simulink model "JT_60SA_scheme_nov_2017_RU_2015a"  (R2015b)
settings: Solver=ode45  SolverMode=SingleTasking  StartTime=startTime-neg_time  StopTime=stopTime  RelTol=1e-5
values from neighbouring files (symbols this model uses):
  A_contr = A    [JT_60SA_simulator_VS_SOF18d66_japs_sensors_adriano_isoflux.m]    (also in JT_60SA_simulator_VS_SOF18d66_japs_sensors_isoflux_sqzd.m)
  B_contr = [B(:,[1:12 end]) A_contr*E]    [JT_60SA_simulator_VS_SOF18d66_japs_sensors_adriano_isoflux.m]    (also in JT_60SA_simulator_VS_SOF18d66_japs_sensors_isoflux_sqzd.m)
  C_contr = LinearModel.C(outputIdx,:)    [JT_60SA_simulator_VS_SOF18d66_japs_sensors_adriano_isoflux.m]    (also in JT_60SA_simulator_VS_SOF18d66_japs_sensors_isoflux_sqzd.m)
  CSsat = [1 1.3 1.3 1] * 1e3    [JT_60SA_simulator_VS_SOF18d66_japs_sensors_adriano_isoflux.m]    (also in JT_60SA_simulator_VS_SOF18d66_japs_sensors_isoflux_sqzd.m)
  D_contr = [LinearModel.D(outputIdx,[1:12 end]) LinearModel.F(outputIdx,:)+C_contr*E]    [JT_60SA_simulator_VS_SOF18d66_japs_sensors_adriano_isoflux.m]    (also in JT_60SA_simulator_VS_SOF18d66_japs_sensors_isoflux_sqzd.m)
  EFsat = [1 .97 .97 .97 .97 1] * 1e3    [JT_60SA_simulator_VS_SOF18d66_japs_sensors_adriano_isoflux.m]    (also in JT_60SA_simulator_VS_SOF18d66_japs_sensors_isoflux_sqzd.m)
  equilDist = LinearModel.YEquil(LinearModel.DisturbancesInfo.OutputPosition)    [JT_60SA_simulator_VS_SOF18d66_japs_sensors_adriano_isoflux.m]    (also in JT_60SA_simulator_VS_SOF18d66_japs_sensors_isoflux_sqzd.m)
  equilOutputs = LinearModel.YEquil(outputIdx)    [JT_60SA_simulator_VS_SOF18d66_japs_sensors_adriano_isoflux.m]    (also in JT_60SA_simulator_VS_SOF18d66_japs_sensors_isoflux_sqzd.m)
  equilVolts = zeros(13,1)    [JT_60SA_simulator_VS_SOF18d66_japs_sensors_adriano_isoflux.m]    (also in JT_60SA_simulator_VS_SOF18d66_japs_sensors_isoflux_sqzd.m)
  I_sat_lower = [-2 -2 -2 -2 -2 -2 -2 -2 -2 -2]*1e4    [JT_60SA_simulator_VS_SOF18d66_japs_sensors_adriano_isoflux.m]    (also in JT_60SA_simulator_VS_SOF18d66_japs_sensors_isoflux_sqzd.m)
  I_sat_upper = [2 2 2 2 1 1 2 2 1 1]*1e4    [JT_60SA_simulator_VS_SOF18d66_japs_sensors_adriano_isoflux.m]    (also in JT_60SA_simulator_VS_SOF18d66_japs_sensors_isoflux_sqzd.m)
  kIp = kIp/norm(kIp)    [JT_60SA_simulator_VS_SOF18d66_japs_sensors_adriano_isoflux.m]    (also in JT_60SA_simulator_VS_SOF18d66_japs_sensors_isoflux_sqzd.m)
  nOfGaps = 85    [JT_60SA_simulator_VS_SOF18d66_japs_sensors_adriano_isoflux.m]    (also in JT_60SA_simulator_VS_SOF18d66_japs_sensors_isoflux_sqzd.m)
  nOfStrikes = 8    [JT_60SA_simulator_VS_SOF18d66_japs_sensors_adriano_isoflux.m]    (also in JT_60SA_simulator_VS_SOF18d66_japs_sensors_isoflux_sqzd.m)
  PSdelay = 1.5e-3    (= 0.0015)    [JT_60SA_simulator_VS_SOF18d66_japs_sensors_adriano_isoflux.m]    (also in JT_60SA_simulator_VS_SOF18d66_japs_sensors_isoflux_sqzd.m)
  PSmodel = tf([1],[PStau 1]) * eye(nPF)    [JT_60SA_simulator_VS_SOF18d66_japs_sensors_adriano_isoflux.m]    (also in JT_60SA_simulator_VS_SOF18d66_japs_sensors_isoflux_sqzd.m)
  vLoop = LinearModel.R(end,end)*Ip0    [JT_60SA_simulator_VS_SOF18d66_japs_sensors_adriano_isoflux.m]    (also in JT_60SA_simulator_VS_SOF18d66_japs_sensors_isoflux_sqzd.m)
  xi0 = zeros(1, size(A_contr, 1))    [JT_60SA_simulator_VS_SOF18d66_japs_sensors_adriano_isoflux.m]    (also in JT_60SA_simulator_VS_SOF18d66_japs_sensors_isoflux_sqzd.m)
  XSC_matrix = XSC_matrix(:, 1:end-1)    [XSC_adriano_isoflux.m]
undefined symbols (not defined in the file or in its folder): KPFcurr, VS
libraries: cstblocks x5
settings Model: Creator=Adriano  LastModifiedBy=Dom
settings DataIOCC: SaveFormat=Array
settings OptimizationCC: BlockReduction=off  BooleanDataType=off
settings DebuggingCC: SaveWithParameterizedLinksMsg=none  UnderspecifiedInitializationDetection=Classic  MergeDetectMultiDrivingBlocksExec=none  SignalResolutionControl=TryResolveAllWithWarning
settings HardwareCC: ProdBitPerPointer=32  ProdLargestAtomicFloat=None  ProdIntDivRoundTo=Undefined  ProdEndianess=Unspecified  ProdWordSize=32  ProdHWDeviceType=32-bit Generic  TargetUnknown=on
settings GRTTargetCC: GeneratePreprocessorConditionals=Disable all
settings ConfigComp: CovModelRefEnable=Off

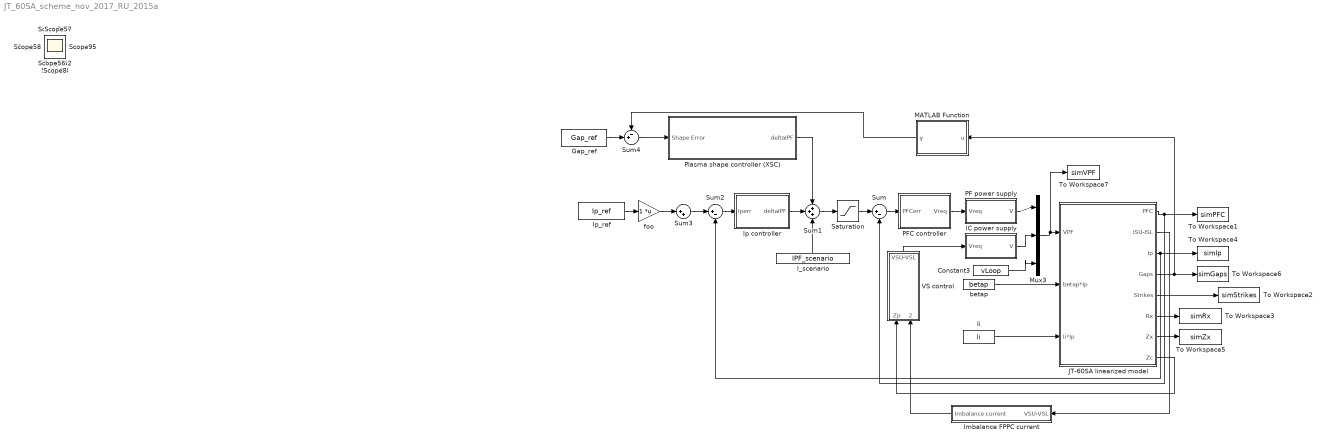
== system JT_60SA_scheme_nov_2017_RU_2015a ==
  Constant3 : Constant  Value=vLoop
  Gap_ref : FromWorkspace  VariableName=Gap_ref  SampleTime=0  OutputAfterFinalValue=Holding final value
  IC power supply : Subsystem
  I_scenario : FromWorkspace  VariableName=IPF_scenario  SampleTime=0  OutputAfterFinalValue=Holding final value
  Imbalance FPPC current : Subsystem
  Ip controller : Subsystem
  Ip_ref : FromWorkspace  VariableName=Ip_ref  SampleTime=0  OutputAfterFinalValue=Holding final value
  JT-60SA linearized model : Subsystem
  MATLAB Function : MATLAB Function  TreatAsAtomicUnit=on
  Mux3 : Mux  Inputs=3
  PF power supply : Subsystem
  PFC controller : Subsystem
  Plasma shape controller (XSC) : Subsystem
  Saturation : Saturate  UpperLimit=I_sat_upper  LowerLimit=I_sat_lower
  Sum : Sum  Inputs=|+-
  Sum1 : Sum  Inputs=+++
  Sum2 : Sum  Inputs=|+-
  Sum3 : Sum  Inputs=|++
  Sum4 : Sum  Inputs=-+|
  To Workspace1 : ToWorkspace  VariableName=simPFC  SaveFormat=Structure With Time  SampleTime=-1
  To Workspace2 : ToWorkspace  VariableName=simStrikes  SaveFormat=Structure With Time  SampleTime=-1
  To Workspace3 : ToWorkspace  VariableName=simRx  SaveFormat=Structure With Time  SampleTime=-1
  To Workspace4 : ToWorkspace  VariableName=simIp  SaveFormat=Structure With Time  SampleTime=-1
  To Workspace5 : ToWorkspace  VariableName=simZx  SaveFormat=Structure With Time  SampleTime=-1
  To Workspace6 : ToWorkspace  VariableName=simGaps  SaveFormat=Structure With Time  SampleTime=-1
  To Workspace7 : ToWorkspace  VariableName=simVPF  SaveFormat=Structure With Time  SampleTime=-1
  VS control : Subsystem
  betap : FromWorkspace  VariableName=betap  SampleTime=0  OutputAfterFinalValue=Holding final value
  foo : Gain  Multiplication=Matrix(K*u)
  li : FromWorkspace  VariableName=li  SampleTime=0  OutputAfterFinalValue=Holding final value
  Scope{,1..58} (59 alike) : Scope
  wires:
  li/1 -> JT-60SA linearized model/3(li*Ip)
  betap/1 -> JT-60SA linearized model/2(betap*Ip)
  JT-60SA linearized model/1(PFC) -> Sum/2, To Workspace1/1
  Mux3/1 -> To Workspace7/1, JT-60SA linearized model/1(VPF)
  Constant3/1 -> Mux3/3
  JT-60SA linearized model/3(Ip) -> To Workspace4/1, Sum2/2
  JT-60SA linearized model/4(Gaps) -> To Workspace6/1, MATLAB Function/1(u)
  JT-60SA linearized model/5(Strikes) -> To Workspace2/1
  JT-60SA linearized model/6(Rx) -> To Workspace3/1
  JT-60SA linearized model/7(Zx) -> To Workspace5/1
  Sum1/1 -> Saturation/1
  PF power supply/1(V) -> Mux3/1
  PFC controller/1(Vreq) -> PF power supply/1(Vreq)
  Sum2/1 -> Ip controller/1(Iperr)
  Sum3/1 -> Sum2/1
  Ip_ref/1 -> foo/1
  foo/1 -> Sum3/1
  Sum4/1 -> Plasma shape controller (XSC)/1(Shape Error)
  Sum/1 -> PFC controller/1(PFCerr)
  Ip controller/1(deltaIPF) -> Sum1/2
  Saturation/1 -> Sum/1
  IC power supply/1(V) -> Mux3/2
  JT-60SA linearized model/8(Zc) -> VS control/1(Zp)
  JT-60SA linearized model/2(ISU-ISL) -> Imbalance FPPC current/1(VSU-VSL)
  Imbalance FPPC current/1(Imbalance current) -> VS control/2(VSU-VSL current)
  VS control/1(VSU-VSL) -> IC power supply/1(Vreq)
  Gap_ref/1 -> Sum4/2
  I_scenario/1 -> Sum1/3
  MATLAB Function/1(y) -> Sum4/1
  Plasma shape controller (XSC)/1(deltaIPF) -> Sum1/1

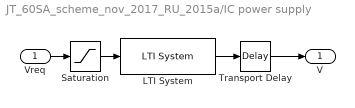
== system JT_60SA_scheme_nov_2017_RU_2015a/IC power supply ==
  Vreq : Inport
  LTI System : cstblocks/LTI System  sys=PSmodel(1:2, 1:2)  IC=[]
  Saturation : Saturate  UpperLimit=[1e3 1e3]  LowerLimit=[-1e3 -1e3]
  Transport Delay : TransportDelay  DelayTime=PSdelay
  V : Outport
  wires:
  LTI System/1 -> Transport Delay/1
  Vreq/1 -> Saturation/1
  Transport Delay/1 -> V/1
  Saturation/1 -> LTI System/1

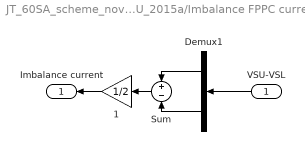
== system JT_60SA_scheme_nov_2017_RU_2015a/Imbalance FPPC current ==
  VSU-VSL : Inport
  "    1" : Gain  Gain=1/2
  Demux1 : Demux  Outputs=2
  Sum : Sum  Inputs=+|-
  Imbalance current : Outport
  wires:
  VSU-VSL/1 -> Demux1/1
  "    1"/1 -> Imbalance current/1
  Demux1/2 -> Sum/2
  Sum/1 -> "    1"/1
  Demux1/1 -> Sum/1

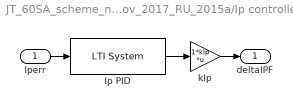
== system JT_60SA_scheme_nov_2017_RU_2015a/Ip controller ==
  Iperr : Inport
  Ip PID : cstblocks/LTI System  sys=Ip_PID  IC=[]
  kIp : Gain  Gain=1*kIp  Multiplication=Matrix(K*u)
  deltaIPF : Outport
  wires:
  Ip PID/1 -> kIp/1
  Iperr/1 -> Ip PID/1
  kIp/1 -> deltaIPF/1

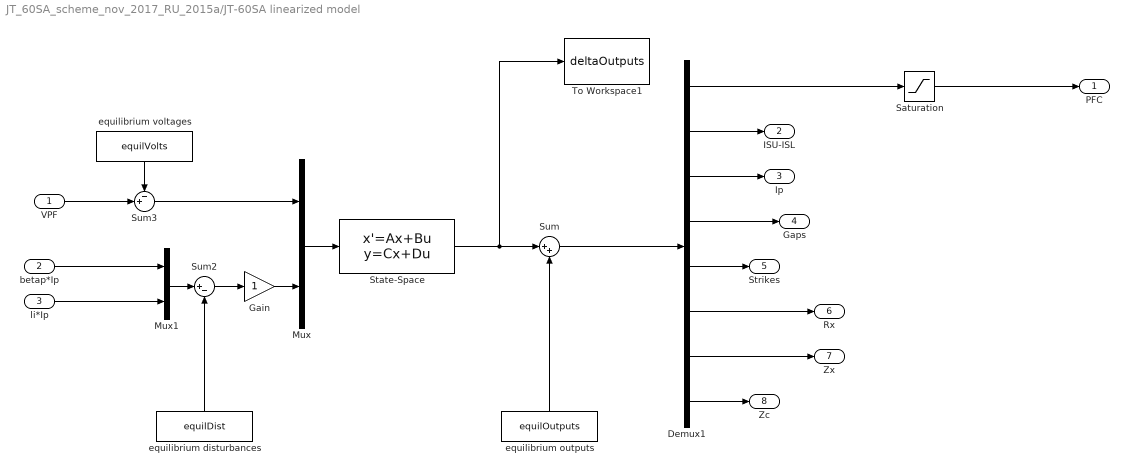
== system JT_60SA_scheme_nov_2017_RU_2015a/JT-60SA linearized model ==
  VPF : Inport
  betap*Ip : Inport  Port=2
  li*Ip : Inport  Port=3
  Demux1 : Demux  Outputs=[10 2 1 nOfGaps nOfStrikes 1 1 1]
  Gain : Gain
  Mux : Mux  Inputs=2
  Mux1 : Mux  Inputs=2
  Saturation : Saturate  UpperLimit=I_sat_upper  LowerLimit=I_sat_lower
  State-Space : StateSpace  A=A_contr  B=B_contr  C=C_contr  D=D_contr  X0=xi0
  Sum : Sum  Inputs=|++
  Sum2 : Sum  Inputs=|+-
  Sum3 : Sum  Inputs=-+|
  To Workspace1 : ToWorkspace  VariableName=deltaOutputs  SaveFormat=Structure With Time  SampleTime=-1
  equilibrium disturbances : Constant  Value=equilDist
  equilibrium outputs : Constant  Value=equilOutputs
  equilibrium voltages : Constant  Value=equilVolts
  PFC : Outport
  ISU-ISL : Outport  Port=2
  Ip : Outport  Port=3
  Gaps : Outport  Port=4
  Strikes : Outport  Port=5
  Rx : Outport  Port=6
  Zx : Outport  Port=7
  Zc : Outport  Port=8
  wires:
  State-Space/1 -> To Workspace1/1, Sum/1
  Sum/1 -> Demux1/1
  equilibrium outputs/1 -> Sum/2
  Mux/1 -> State-Space/1
  VPF/1 -> Sum3/2
  Demux1/1 -> Saturation/1
  Mux1/1 -> Sum2/1
  equilibrium disturbances/1 -> Sum2/2
  betap*Ip/1 -> Mux1/1
  li*Ip/1 -> Mux1/2
  Sum3/1 -> Mux/1
  equilibrium voltages/1 -> Sum3/1
  Sum2/1 -> Gain/1
  Demux1/3 -> Ip/1
  Demux1/4 -> Gaps/1
  Demux1/5 -> Strikes/1
  Demux1/6 -> Rx/1
  Demux1/7 -> Zx/1
  Gain/1 -> Mux/2
  Saturation/1 -> PFC/1
  Demux1/2 -> ISU-ISL/1
  Demux1/8 -> Zc/1

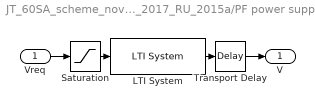
== system JT_60SA_scheme_nov_2017_RU_2015a/PF power supply ==
  Vreq : Inport
  LTI System : cstblocks/LTI System  sys=PSmodel  IC=[]
  Saturation : Saturate  UpperLimit=[CSsat EFsat]  LowerLimit=-[CSsat EFsat]
  Transport Delay : TransportDelay  DelayTime=PSdelay
  V : Outport
  wires:
  LTI System/1 -> Transport Delay/1
  Vreq/1 -> Saturation/1
  Transport Delay/1 -> V/1
  Saturation/1 -> LTI System/1

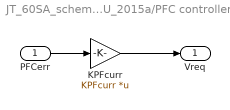
== system JT_60SA_scheme_nov_2017_RU_2015a/PFC controller ==
  PFCerr : Inport
  KPFcurr : Gain  Gain=KPFcurr  Multiplication=Matrix(K*u)
  Vreq : Outport
  wires:
  KPFcurr/1 -> Vreq/1
  PFCerr/1 -> KPFcurr/1

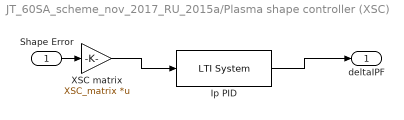
== system JT_60SA_scheme_nov_2017_RU_2015a/Plasma shape controller (XSC) ==
  Shape Error : Inport
  Ip PID : cstblocks/LTI System  sys=XSC_PI  IC=[]
  XSC matrix : Gain  Gain=XSC_matrix  Multiplication=Matrix(K*u)
  deltaIPF : Outport
  wires:
  Shape Error/1 -> XSC matrix/1
  XSC matrix/1 -> Ip PID/1
  Ip PID/1 -> deltaIPF/1

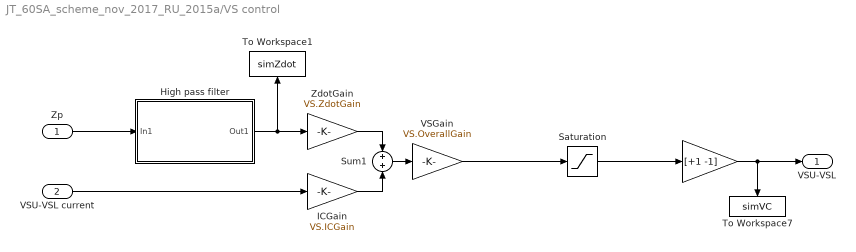
== system JT_60SA_scheme_nov_2017_RU_2015a/VS control ==
  Zp : Inport
  VSU-VSL current : Inport  Port=2
  "    " : Gain  Gain=[+1 -1]
  High pass filter : Subsystem
  ICGain : Gain  Gain=VS.ICGain
  Saturation : Saturate  UpperLimit=1e3  LowerLimit=-1e3
  Sum1 : Sum  Inputs=+|+
  To Workspace1 : ToWorkspace  VariableName=simZdot  SaveFormat=Structure With Time  SampleTime=-1
  To Workspace7 : ToWorkspace  VariableName=simVC  SaveFormat=Structure With Time  SampleTime=-1
  VSGain : Gain  Gain=VS.OverallGain
  ZdotGain : Gain  Gain=VS.ZdotGain
  VSU-VSL : Outport
  wires:
  VSU-VSL current/1 -> ICGain/1
  High pass filter/1(Out1) -> To Workspace1/1, ZdotGain/1
  Zp/1 -> High pass filter/1(In1)
  Sum1/1 -> VSGain/1
  ZdotGain/1 -> Sum1/1
  ICGain/1 -> Sum1/2
  "    "/1 -> VSU-VSL/1, To Workspace7/1
  VSGain/1 -> Saturation/1
  Saturation/1 -> "    "/1

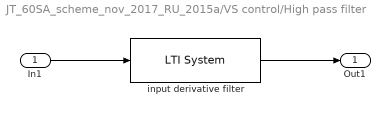
== system JT_60SA_scheme_nov_2017_RU_2015a/VS control/High pass filter ==
  In1 : Inport
  input derivative filter : cstblocks/LTI System  sys=VS.Filter  IC=[]
  Out1 : Outport
  wires:
  input derivative filter/1 -> Out1/1
  In1/1 -> input derivative filter/1

== matlab function JT_60SA_scheme_nov_2017_RU_2015a/MATLAB Function ==
  data: u input; y output
function y = fcn(u)
%#codegen
% % % %%all gaps
% y=u(1:end);

% %%30 gaps
%  y=u([1:3:(end-2),end-1,end]);
    
% %%19 gaps
%  y=u([1:5:(end-2),end-1,end]);

%20 gaps
 y=u([round((1+1:4.6:(end-2))),end-1,end]);

% % % Japanese selection1
% japs_gaps=[13,22,36,52,66,76,84,85  ]';
%  y=u(japs_gaps);
% % % % % % 
% % % %Japanese selection 2
%  japs_gaps=[21,36,47,66,84,85]';
% y=u(japs_gaps);

%
